simulink model "Squelette_DSPBuilder_ModulateurOQPSK"  (R2016a)
settings: Solver=FixedStepDiscrete  StartTime=0.0  StopTime=1e-3/500  RelTol=1e-3
InitFcn:
  | %% DSPBuilder Start
  | alt_dspbuilder_update_model(bdroot)
  | %% DSPBuilder End
libraries: allblocks_alteradspbuilder2 x84
settings Model: Creator=rhev2401  LastModifiedBy=dufd2703
settings DataIOCC: LimitDataPoints=on  SaveFormat=Array  SignalLoggingSaveFormat=ModelDataLogs
settings DebuggingCC: SolverPrmCheckMsg=warning  MultiTaskDSMMsg=warning  MultiTaskCondExecSysMsg=none
settings HardwareCC: ProdBitPerPointer=32  ProdLargestAtomicFloat=None  ProdIntDivRoundTo=Undefined  ProdEndianess=Unspecified  ProdWordSize=32  ProdHWDeviceType=32-bit Generic
settings ModelReferenceCC: PropagateSignalLabelsOutOfModel=off
settings ConfigComp: CovModelRefEnable=Off  CovSFcnEnable=off

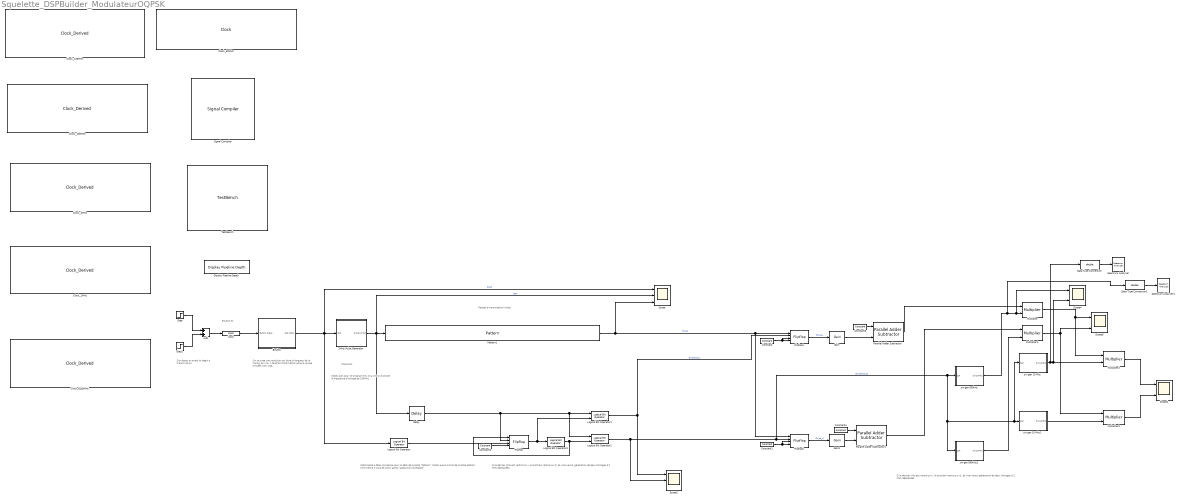
== system Squelette_DSPBuilder_ModulateurOQPSK ==
  note: Simulates an event to begin a transmission
  note: Bouton 01
  note: On se crée une impulsion qui dure la longueur de la trame.
      |
      | En vrai, il faudrait transmettre jusqu'à ce que le buffer soit vide...
  note: Paquet à transmettre (chips)
  note: Chipclock
  note: Notez que, pour ce programme, on a choisi d'utiliser la fréquence d'horloge de 100MHz.
  note: Si le dernier chip est rentré sur I, le prochain rentre sur Q, et vice-versa; génération de deux horloges d'1 MHz déphasées
  note: Cette boîte à délai compense pour le délai de la boîte "Pattern" (notez que la sortie de la boîte pattern commence 1 coup de clock après l'apparition du Enable)
  note: Si le dernier chip est rentré sur I, le prochain rentre sur Q, et vice-versa; génération de deux horloges d'1 MHz déphasées
  2MHz Pulse Generator : Subsystem
  Add : Sum
  Bouton : Subsystem
  Clock_100MHz : allblocks_alteradspbuilder2/Clock_Derived  ClockNumerator=1  ClockDenominator=2  ResetLatency=0  ResetRegisterCascadeDepth=0  SimulationStartCycle=5  PhaseOffset=0  Reset=aclr_100MHz  ResetType=Active Low  Export=off
  Clock_125MHz : allblocks_alteradspbuilder2/Clock_Derived  ClockNumerator=10  ClockDenominator=25  ResetLatency=0  ResetRegisterCascadeDepth=0  SimulationStartCycle=5  PhaseOffset=0  Reset=aclr_125MHz  ResetType=Active Low  Export=off
  Clock_1MHz : allblocks_alteradspbuilder2/Clock_Derived  ClockNumerator=50  ClockDenominator=1  ResetLatency=0  ResetRegisterCascadeDepth=0  SimulationStartCycle=5  PhaseOffset=0  Reset=aclr_1MHz  ResetType=Active Low  Export=off
  Clock_2MHz : allblocks_alteradspbuilder2/Clock_Derived  ClockNumerator=25  ClockDenominator=1  ResetLatency=0  ResetRegisterCascadeDepth=0  SimulationStartCycle=5  PhaseOffset=0  Reset=aclr_2MHz  ResetType=Active Low  Export=off
  Clock_50MHz : allblocks_alteradspbuilder2/Clock  ClockPeriod=20  ClockPeriodUnit=ns  SampleTime=20e-9  ResetLatency=0  ResetRegisterCascadeDepth=0  SimulationStartCycle=5  PhaseOffset=0  Reset=aclr  ResetType=Active Low  Export=off
  Clock_62p5MHz : allblocks_alteradspbuilder2/Clock_Derived  ClockNumerator=800  ClockDenominator=1  ResetLatency=0  ResetRegisterCascadeDepth=0  SimulationStartCycle=5  PhaseOffset=0  Reset=aclr_62p5MHz  ResetType=Active Low  Export=off
  Constant : allblocks_alteradspbuilder2/Constant  mask_cst=1  BusType=Signed Integer  bwl=8  bwr=0  roundMode=Truncate  satMode=Wrap  SpecifyClock=off  allowFloatingPointOverride=on  logOutputs=off  logFile=U:\projet-s6\DSP builder\Squelette_ModulateurOQPSK\tb_Squelette_DSPBuilder_ModulateurOQPSK\Squelette%5FDSPBuilder%5FModulateurOQPSK_Constant.fixedpointlog
  Constant1 : allblocks_alteradspbuilder2/Constant  mask_cst=1  BusType=Signed Integer  bwl=8  bwr=0  roundMode=Truncate  satMode=Wrap  SpecifyClock=off  allowFloatingPointOverride=on  logOutputs=off  logFile=U:\projet-s6\DSP builder\Squelette_ModulateurOQPSK\tb_Squelette_DSPBuilder_ModulateurOQPSK\Squelette%5FDSPBuilder%5FModulateurOQPSK_Constant1.fixedpointlog
  Constant2 : allblocks_alteradspbuilder2/Constant  mask_cst=1  BusType=Signed Integer  bwl=8  bwr=0  roundMode=Truncate  satMode=Wrap  SpecifyClock=off  allowFloatingPointOverride=on  logOutputs=off  logFile=U:\projet-s6\DSP builder\Squelette_ModulateurOQPSK\tb_Squelette_DSPBuilder_ModulateurOQPSK\Squelette%5FDSPBuilder%5FModulateurOQPSK_Constant2.fixedpointlog
  Constant3 : allblocks_alteradspbuilder2/Constant  mask_cst=1  BusType=Unsigned Integer  bwl=1  bwr=0  roundMode=Truncate  satMode=Wrap  SpecifyClock=off  allowFloatingPointOverride=on  logOutputs=off  logFile=U:\projet-s6\DSP builder\Squelette_ModulateurOQPSK\tb_Squelette_DSPBuilder_ModulateurOQPSK\Squelette%5FDSPBuilder%5FModulateurOQPSK_Constant3.fixedpointlog
  Constant4 : allblocks_alteradspbuilder2/Constant  mask_cst=1  BusType=Unsigned Integer  bwl=1  bwr=0  roundMode=Truncate  satMode=Wrap  SpecifyClock=off  allowFloatingPointOverride=on  logOutputs=off  logFile=U:\projet-s6\DSP builder\Squelette_ModulateurOQPSK\tb_Squelette_DSPBuilder_ModulateurOQPSK\Squelette%5FDSPBuilder%5FModulateurOQPSK_Constant4.fixedpointlog
  Data Type Conversion : DataTypeConversion  OutDataTypeStr=double
  Data Type Conversion1 : DataTypeConversion  OutDataTypeStr=double
  Delay : allblocks_alteradspbuilder2/Delay  pipeline=1  pipeline_display=1  ClockPhase=1  use_ena=off  use_sclr=off  allowFloatingPointOverride=on  logOutputs=off  logFile=U:\projet-s6\DSP builder\Squelette_ModulateurOQPSK\tb_Squelette_DSPBuilder_ModulateurOQPSK\Squelette%5FDSPBuilder%5FModulateurOQPSK_Delay.fixedpointlog  use_init=off  reset_value=1
  Display Pipeline Depth : allblocks_alteradspbuilder2/Display Pipeline Depth  DisplayLatencyOnBlocks=on
  Flipflop : allblocks_alteradspbuilder2/Flipflop  mode=DFFE  BusType=Single Bit  bwl=2  bwr=2  pipeline_display=1
  Flipflop1 : allblocks_alteradspbuilder2/Flipflop  mode=DFFE  BusType=Single Bit  bwl=2  bwr=2  pipeline_display=1
  Flipflop2 : allblocks_alteradspbuilder2/Flipflop  mode=DFFE  BusType=Single Bit  bwl=2  bwr=2  pipeline_display=1
  Gain : allblocks_alteradspbuilder2/Gain  vgain=2  BusType=Signed Integer  bwl=3  bwr=0  pipeline=1  pipeline_display=1  allowFloatingPointOverride=on  logOutputs=off  logFile=U:\projet-s6\DSP builder\Squelette_ModulateurOQPSK\tb_Squelette_DSPBuilder_ModulateurOQPSK\Squelette%5FDSPBuilder%5FModulateurOQPSK_Gain.fixedpointlog  use_ena=off  use_aclr=off  lpm=off  MaskValue=1
  Gain1 : allblocks_alteradspbuilder2/Gain  vgain=2  BusType=Signed Integer  bwl=3  bwr=0  pipeline=1  pipeline_display=1  allowFloatingPointOverride=on  logOutputs=off  logFile=U:\projet-s6\DSP builder\Squelette_ModulateurOQPSK\tb_Squelette_DSPBuilder_ModulateurOQPSK\Squelette%5FDSPBuilder%5FModulateurOQPSK_Gain1.fixedpointlog  use_ena=off  use_aclr=off  lpm=off  MaskValue=1
  Input : allblocks_alteradspbuilder2/Input  iofile=U:\projet-s6\DSP builder\Squelette_ModulateurOQPSK\tb_Squelette_DSPBuilder_ModulateurOQPSK\Squelette%5FDSPBuilder%5FModulateurOQPSK_Input.salt  BusType=Single Bit  bwl=1  bwr=0  SpecifyClock=on  clock=Clock_100MHz  PORTTYPE=Input  externalType=Inferred  allowFloatingPointOverride=on  logOutputs=off
  Logical Bit Operator : allblocks_alteradspbuilder2/Logical Bit Operator  LogicalOperator=NOT  user_inputs=2  pipeline_display=0
  Logical Bit Operator1 : allblocks_alteradspbuilder2/Logical Bit Operator  LogicalOperator=AND  user_inputs=2  pipeline_display=0
  Logical Bit Operator2 : allblocks_alteradspbuilder2/Logical Bit Operator  LogicalOperator=AND  user_inputs=2  pipeline_display=0
  Logical Bit Operator3 : allblocks_alteradspbuilder2/Logical Bit Operator  LogicalOperator=NOT  user_inputs=2  pipeline_display=0
  Multiplier : allblocks_alteradspbuilder2/Multiplier  BusType=Signed Integer  bwl=6  bwr=0  pipeline=0  pipeline_display=0  allowFloatingPointOverride=on  logOutputs=off  logFile=U:\projet-s6\DSP builder\Squelette_ModulateurOQPSK\tb_Squelette_DSPBuilder_ModulateurOQPSK\Squelette%5FDSPBuilder%5FModulateurOQPSK_Multiplier.fixedpointlog  UseEqualInputWidth=off  bbwl=14  bbwr=0  FullResolution=on  OutputMsb=8  OutputLsb=0  OutputBwl=16  OutputBwr=16  UseDedicatedCircuitry=YES  use_ena=off  use_aclr=off
  Multiplier1 : allblocks_alteradspbuilder2/Multiplier  BusType=Signed Integer  bwl=6  bwr=0  pipeline=0  pipeline_display=0  allowFloatingPointOverride=on  logOutputs=off  logFile=U:\projet-s6\DSP builder\Squelette_ModulateurOQPSK\tb_Squelette_DSPBuilder_ModulateurOQPSK\Squelette%5FDSPBuilder%5FModulateurOQPSK_Multiplier1.fixedpointlog  UseEqualInputWidth=off  bbwl=14  bbwr=0  FullResolution=on  OutputMsb=8  OutputLsb=0  OutputBwl=16  OutputBwr=16  UseDedicatedCircuitry=YES  use_ena=off  use_aclr=off
  Multiplier2 : allblocks_alteradspbuilder2/Multiplier  BusType=Signed Integer  bwl=16  bwr=0  pipeline=0  pipeline_display=0  allowFloatingPointOverride=on  logOutputs=off  logFile=U:\projet-s6\DSP builder\Squelette_ModulateurOQPSK\tb_Squelette_DSPBuilder_ModulateurOQPSK\Squelette%5FDSPBuilder%5FModulateurOQPSK_Multiplier2.fixedpointlog  UseEqualInputWidth=off  bbwl=14  bbwr=0  FullResolution=on  OutputMsb=8  OutputLsb=0  OutputBwl=16  OutputBwr=16  UseDedicatedCircuitry=YES  use_ena=off  use_aclr=off
  Multiplier3 : allblocks_alteradspbuilder2/Multiplier  BusType=Signed Integer  bwl=16  bwr=0  pipeline=0  pipeline_display=0  allowFloatingPointOverride=on  logOutputs=off  logFile=U:\projet-s6\DSP builder\Squelette_ModulateurOQPSK\tb_Squelette_DSPBuilder_ModulateurOQPSK\Squelette%5FDSPBuilder%5FModulateurOQPSK_Multiplier3.fixedpointlog  UseEqualInputWidth=off  bbwl=14  bbwr=0  FullResolution=on  OutputMsb=8  OutputLsb=0  OutputBwl=16  OutputBwr=16  UseDedicatedCircuitry=YES  use_ena=off  use_aclr=off
  Parallel Adder Subtractor : allblocks_alteradspbuilder2/Parallel Adder Subtractor  number_of_inputs=2  direction=-+  use_pipeline=off  pipeline_display=0  phase_selection=1  use_ena=off  use_aclr=off  allowFloatingPointOverride=on  logOutputs=off  logFile=U:\projet-s6\DSP builder\Squelette_ModulateurOQPSK\tb_Squelette_DSPBuilder_ModulateurOQPSK\Squelette%5FDSPBuilder%5FModulateurOQPSK_Parallel+Adder+Subtractor.fixedpointlog
  Parallel Adder Subtractor1 : allblocks_alteradspbuilder2/Parallel Adder Subtractor  number_of_inputs=2  direction=-+  use_pipeline=off  pipeline_display=0  phase_selection=1  use_ena=off  use_aclr=off  allowFloatingPointOverride=on  logOutputs=off  logFile=U:\projet-s6\DSP builder\Squelette_ModulateurOQPSK\tb_Squelette_DSPBuilder_ModulateurOQPSK\Squelette%5FDSPBuilder%5FModulateurOQPSK_Parallel+Adder+Subtractor1.fixedpointlog
  Pattern1 : allblocks_alteradspbuilder2/Pattern  Sequence=10011010111100001100110000110011  SpecifyClock=off  clock=Clock_250kHz  use_ena=on  use_sclr=off
  Scope : Scope  NumInputPorts=3
  Scope1 : Scope  NumInputPorts=2
  Scope2 : Scope  NumInputPorts=3
  Scope3 : Scope  NumInputPorts=2
  Scope4 : Scope  NumInputPorts=2
  Signal Compiler : allblocks_alteradspbuilder2/Signal Compiler  DeviceFamily=Cyclone V  DeviceName=AUTO  DisableEarlyHDLGeneration=off  EnableSignalTap=off  SignalTapDepth=128  UseBoardBlock=off  StpUseDefaultClock=on  StpClock=Clock_50MHz  ExportDir=C:\Users\pivd2501\Documents  MAX10_ProgrammingMode=Internal Flash (SDM) Single Boot
  Spectrum Analyzer : SpectrumAnalyzer
  Spectrum Analyzer1 : SpectrumAnalyzer
  Step : Step  Time=100e-6  Before=1  After=0  SampleTime=1/100e06  VectorParams1D=off
  Step1 : Step  Time=200e-6  SampleTime=1/100e06  VectorParams1D=off
  TestBench : allblocks_alteradspbuilder2/TestBench  enable=on  advancedMode=on  modelSimGui=on  maxDisplayErrors=1000  mismatchErrorLevel=Error  simdatafile=U:\projet-s6\DSP builder\Squelette_ModulateurOQPSK\tb_Squelette_DSPBuilder_ModulateurOQPSK\Squelette_DSPBuilder_ModulateurOQPSK.simdata.tcl
  sin gen 10 Mhz : Subsystem
  sin gen 10 Mhz1 : Subsystem
  sin gen 500kHz : Subsystem
  sin gen 500kHz2 : Subsystem
  wires:
  Add/1 -> Input/1
  Step1/1 -> Add/2
  Step/1 -> Add/1
  2MHz Pulse Generator/1(Pulse 2MHz) -> Delay/1, Pattern1/1, Scope/2  "ENA"
  Pattern1/1 -> Flipflop2/1, Flipflop1/1, Scope/3  "Chips"
  Bouton/1(CLR 480u) -> Logical Bit Operator/1, 2MHz Pulse Generator/1(CLR), Scope/1  "SCLR"
  Input/1 -> Bouton/1(Button Press)
  Flipflop/1 -> Logical Bit Operator1/2, Logical Bit Operator3/1
  Logical Bit Operator3/1 -> Flipflop/1, Logical Bit Operator2/2
  Logical Bit Operator1/1 -> Scope2/1, Flipflop1/2  "ChipClock_I"
  Constant/1 -> Flipflop1/4, Flipflop1/3
  Constant1/1 -> Flipflop2/3, Flipflop2/4
  Logical Bit Operator2/1 -> Scope2/2, sin gen 10 Mhz/1(CLR), sin gen 10 Mhz1/1(CLR), sin gen 500kHz2/1(CLR), sin gen 500kHz/1(CLR), Flipflop2/2  "ChipClock_Q"
  Logical Bit Operator/1 -> Flipflop/3
  Constant2/1 -> Flipflop/4
  Delay/1 -> Flipflop/2, Logical Bit Operator2/1, Logical Bit Operator1/1
  sin gen 500kHz/1(Sin10Mhz) -> Data Type Conversion1/1, Scope4/1, Multiplier/2
  sin gen 500kHz2/1(Sin10Mhz) -> Multiplier1/2
  Multiplier/1 -> Scope3/1, Multiplier2/1
  Multiplier1/1 -> Multiplier3/1, Scope3/2
  sin gen 10 Mhz/1(Sin10Mhz) -> Data Type Conversion/1, Scope4/2, Multiplier2/2
  sin gen 10 Mhz1/1(Sin10Mhz) -> Multiplier3/2
  Multiplier2/1 -> Scope1/1
  Multiplier3/1 -> Scope1/2
  Flipflop1/1 -> Gain/1  "Chips_I"
  Parallel Adder Subtractor/1 -> Multiplier/1
  Constant3/1 -> Parallel Adder Subtractor/1
  Gain/1 -> Parallel Adder Subtractor/2
  Flipflop2/1 -> Gain1/1  "Chips_Q"
  Gain1/1 -> Parallel Adder Subtractor1/2
  Constant4/1 -> Parallel Adder Subtractor1/1
  Parallel Adder Subtractor1/1 -> Multiplier1/1
  Data Type Conversion/1 -> Spectrum Analyzer/1
  Data Type Conversion1/1 -> Spectrum Analyzer1/1

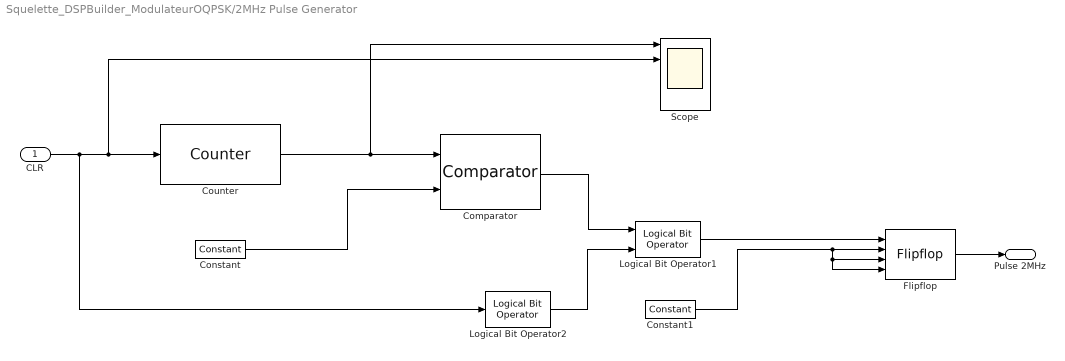
== system Squelette_DSPBuilder_ModulateurOQPSK/2MHz Pulse Generator ==
  CLR : Inport
  Comparator : allblocks_alteradspbuilder2/Comparator  direction=a == b  pipeline_display=0  allowFloatingPointOverride=on  logOutputs=off  logFile=U:\projet-s6\DSP builder\Squelette_ModulateurOQPSK\tb_Squelette_DSPBuilder_ModulateurOQPSK\Squelette%5FDSPBuilder%5FModulateurOQPSK_2MHz+Pulse+Generator_Comparator.fixedpointlog
  Constant : allblocks_alteradspbuilder2/Constant  mask_cst=0  BusType=Unsigned Integer  bwl=1  bwr=0  roundMode=Truncate  satMode=Wrap  SpecifyClock=off  allowFloatingPointOverride=on  logOutputs=off  logFile=U:\projet-s6\DSP builder\Squelette_ModulateurOQPSK\tb_Squelette_DSPBuilder_ModulateurOQPSK\Squelette%5FDSPBuilder%5FModulateurOQPSK_2MHz+Pulse+Generator_Constant.fixedpointlog
  Constant1 : allblocks_alteradspbuilder2/Constant  mask_cst=1  BusType=Unsigned Integer  bwl=1  bwr=0  roundMode=Truncate  satMode=Wrap  SpecifyClock=off  allowFloatingPointOverride=on  logOutputs=off  logFile=U:\projet-s6\DSP builder\Squelette_ModulateurOQPSK\tb_Squelette_DSPBuilder_ModulateurOQPSK\Squelette%5FDSPBuilder%5FModulateurOQPSK_2MHz+Pulse+Generator_Constant1.fixedpointlog
  Counter : allblocks_alteradspbuilder2/Counter  BusType=Unsigned Integer  bwl=10  bwr=0  use_modulo=on  modulo=50  SpecifyClock=off  direction=Increment  use_sload=off  use_sset=off  svalue=1  use_clk_ena=off  use_ena=off  use_sclr=on  pipeline_display=1
  Flipflop : allblocks_alteradspbuilder2/Flipflop  mode=DFFE  BusType=Single Bit  bwl=2  bwr=2  pipeline_display=1
  Logical Bit Operator1 : allblocks_alteradspbuilder2/Logical Bit Operator  LogicalOperator=AND  user_inputs=2  pipeline_display=0
  Logical Bit Operator2 : allblocks_alteradspbuilder2/Logical Bit Operator  LogicalOperator=NOT  user_inputs=2  pipeline_display=0
  Scope : Scope  NumInputPorts=5
  Pulse 2MHz : Outport
  wires:
  Counter/1 -> Scope/1, Comparator/1
  Constant/1 -> Comparator/2
  CLR/1 -> Logical Bit Operator2/1, Scope/2, Counter/1
  Logical Bit Operator2/1 -> Logical Bit Operator1/2
  Comparator/1 -> Logical Bit Operator1/1
  Flipflop/1 -> Pulse 2MHz/1
  Logical Bit Operator1/1 -> Flipflop/1
  Constant1/1 -> Flipflop/4, Flipflop/3, Flipflop/2

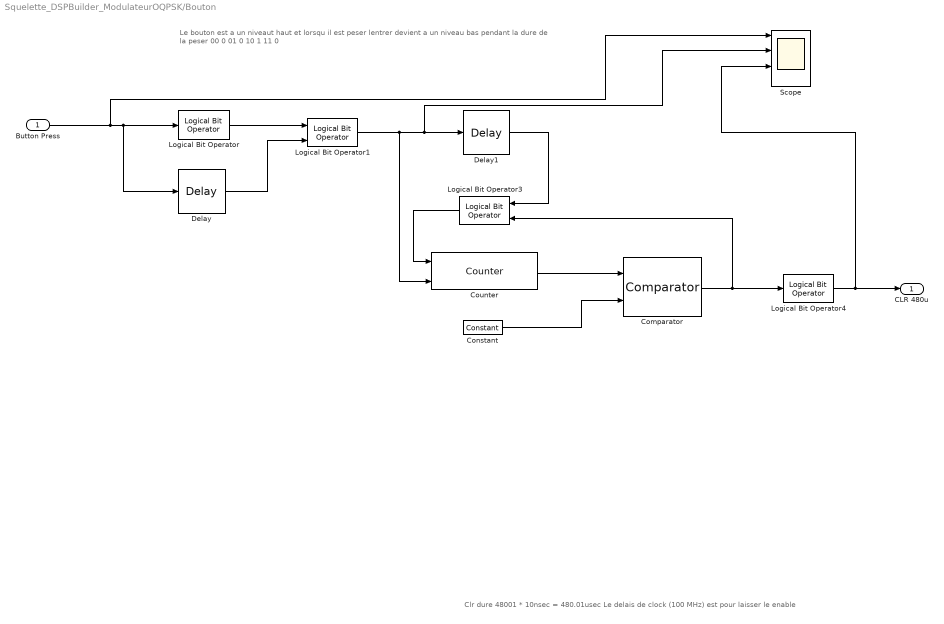
== system Squelette_DSPBuilder_ModulateurOQPSK/Bouton ==
  note: Clr dure 48001 * 10nsec = 480.01usec Le delais de clock (100 MHz) est pour laisser le enable
  note: Le bouton est a un niveaut haut et lorsqu il est peser lentrer devient a un niveau bas pendant la dure de la peser
      |
      | 00  0
      | 01  0
      | 10  1
      | 11  0
  Button Press : Inport
  Comparator : allblocks_alteradspbuilder2/Comparator  direction=a >= b  pipeline_display=0  allowFloatingPointOverride=on  logOutputs=off  logFile=U:\projet-s6\DSP builder\Squelette_ModulateurOQPSK\tb_Squelette_DSPBuilder_ModulateurOQPSK\Squelette%5FDSPBuilder%5FModulateurOQPSK_Bouton_Comparator.fixedpointlog
  Constant : allblocks_alteradspbuilder2/Constant  mask_cst=1  BusType=Unsigned Integer  bwl=8  bwr=0  roundMode=Truncate  satMode=Wrap  SpecifyClock=off  allowFloatingPointOverride=on  logOutputs=off  logFile=U:\projet-s6\DSP builder\Squelette_ModulateurOQPSK\tb_Squelette_DSPBuilder_ModulateurOQPSK\Squelette%5FDSPBuilder%5FModulateurOQPSK_Bouton_Constant.fixedpointlog
  Counter : allblocks_alteradspbuilder2/Counter  BusType=Unsigned Integer  bwl=16  bwr=0  use_modulo=on  modulo=48001  SpecifyClock=off  clock=Clock_100MHz  direction=Increment  use_sload=off  use_sset=off  svalue=1  use_clk_ena=off  use_ena=on  use_sclr=on  pipeline_display=1
  Delay : allblocks_alteradspbuilder2/Delay  pipeline=1  pipeline_display=1  ClockPhase=1  use_ena=off  use_sclr=off  allowFloatingPointOverride=on  logOutputs=off  logFile=U:\projet-s6\DSP builder\Squelette_ModulateurOQPSK\tb_Squelette_DSPBuilder_ModulateurOQPSK\Squelette%5FDSPBuilder%5FModulateurOQPSK_Bouton_Delay.fixedpointlog  use_init=off  reset_value=1
  Delay1 : allblocks_alteradspbuilder2/Delay  pipeline=1  pipeline_display=1  ClockPhase=1  use_ena=off  use_sclr=off  allowFloatingPointOverride=on  logOutputs=off  logFile=U:\projet-s6\DSP builder\Squelette_ModulateurOQPSK\tb_Squelette_DSPBuilder_ModulateurOQPSK\Squelette%5FDSPBuilder%5FModulateurOQPSK_Bouton_Delay1.fixedpointlog  use_init=off  reset_value=1
  Logical Bit Operator : allblocks_alteradspbuilder2/Logical Bit Operator  LogicalOperator=NOT  user_inputs=2  pipeline_display=0
  Logical Bit Operator1 : allblocks_alteradspbuilder2/Logical Bit Operator  LogicalOperator=AND  user_inputs=2  pipeline_display=0
  Logical Bit Operator3 : allblocks_alteradspbuilder2/Logical Bit Operator  LogicalOperator=OR  user_inputs=2  pipeline_display=0
  Logical Bit Operator4 : allblocks_alteradspbuilder2/Logical Bit Operator  LogicalOperator=NOT  user_inputs=2  pipeline_display=0
  Scope : Scope  NumInputPorts=4
  CLR 480u : Outport
  wires:
  Button Press/1 -> Scope/1, Logical Bit Operator/1, Delay/1
  Logical Bit Operator/1 -> Logical Bit Operator1/1
  Logical Bit Operator1/1 -> Scope/2, Delay1/1, Counter/2
  Counter/1 -> Comparator/1
  Constant/1 -> Comparator/2
  Delay1/1 -> Logical Bit Operator3/1
  Logical Bit Operator3/1 -> Counter/1
  Comparator/1 -> Logical Bit Operator3/2, Logical Bit Operator4/1
  Delay/1 -> Logical Bit Operator1/2
  Logical Bit Operator4/1 -> Scope/3, CLR 480u/1

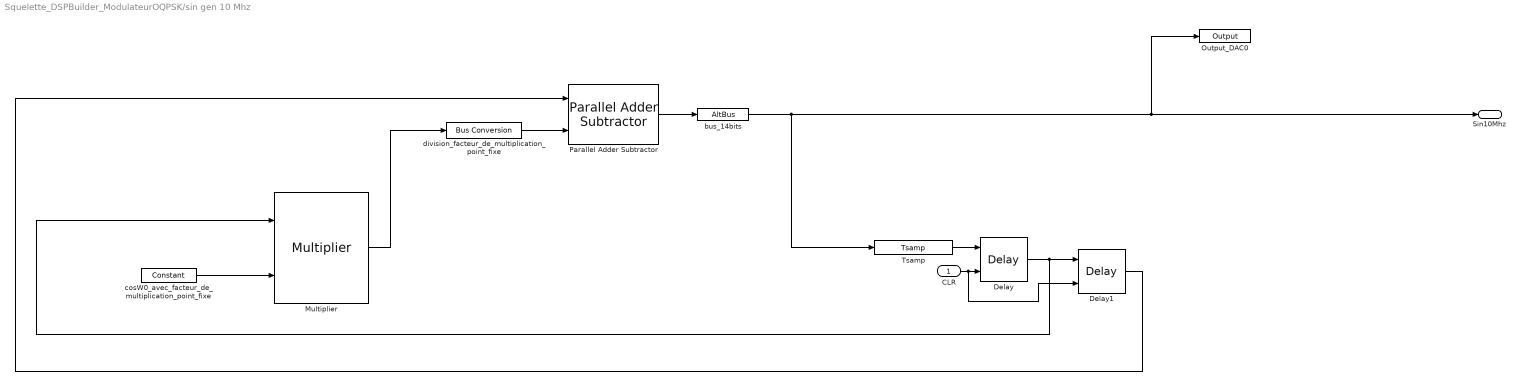
== system Squelette_DSPBuilder_ModulateurOQPSK/sin gen 10 Mhz ==
  CLR : Inport
  Delay : allblocks_alteradspbuilder2/Delay  pipeline=1  pipeline_display=1  ClockPhase=1  use_ena=off  use_sclr=on  allowFloatingPointOverride=on  logOutputs=off  logFile=U:\projet-s6\DSP builder\Squelette_ModulateurOQPSK\tb_Squelette_DSPBuilder_ModulateurOQPSK\Squelette%5FDSPBuilder%5FModulateurOQPSK_sin+gen+10+Mhz_Delay.fixedpointlog  use_init=on  reset_value=y_n_1_10M
  Delay1 : allblocks_alteradspbuilder2/Delay  pipeline=1  pipeline_display=1  ClockPhase=1  use_ena=off  use_sclr=on  allowFloatingPointOverride=on  logOutputs=off  logFile=U:\projet-s6\DSP builder\Squelette_ModulateurOQPSK\tb_Squelette_DSPBuilder_ModulateurOQPSK\Squelette%5FDSPBuilder%5FModulateurOQPSK_sin+gen+10+Mhz_Delay1.fixedpointlog  use_init=on  reset_value=y_n_2_10M
  Multiplier : allblocks_alteradspbuilder2/Multiplier  BusType=Signed Integer  bwl=14  bwr=0  pipeline=0  pipeline_display=0  allowFloatingPointOverride=on  logOutputs=off  logFile=U:\projet-s6\DSP builder\Squelette_ModulateurOQPSK\tb_Squelette_DSPBuilder_ModulateurOQPSK\Squelette%5FDSPBuilder%5FModulateurOQPSK_sin+gen+10+Mhz_Multiplier.fixedpointlog  UseEqualInputWidth=off  bbwl=19  bbwr=0  FullResolution=on  OutputMsb=8  OutputLsb=0  OutputBwl=16  OutputBwr=16  UseDedicatedCircuitry=YES  use_ena=off  use_aclr=off
  Output_DAC0 : allblocks_alteradspbuilder2/Output  iofile=U:\projet-s6\DSP builder\Squelette_ModulateurOQPSK\tb_Squelette_DSPBuilder_ModulateurOQPSK\Squelette%5FDSPBuilder%5FModulateurOQPSK_sin+gen+10+Mhz_Output%5FDAC0.capture  BusType=Signed Integer  bwl=14  bwr=0  externalType=Inferred  PORTTYPE=Output  allowFloatingPointOverride=on  logOutputs=off
  Parallel Adder Subtractor : allblocks_alteradspbuilder2/Parallel Adder Subtractor  number_of_inputs=2  direction=-+  use_pipeline=off  pipeline_display=0  phase_selection=1  use_ena=off  use_aclr=off  allowFloatingPointOverride=on  logOutputs=off  logFile=U:\projet-s6\DSP builder\Squelette_ModulateurOQPSK\tb_Squelette_DSPBuilder_ModulateurOQPSK\Squelette%5FDSPBuilder%5FModulateurOQPSK_sin+gen+10+Mhz_Parallel+Adder+Subtractor.fixedpointlog
  Tsamp : allblocks_alteradspbuilder2/Tsamp  SpecifyClock=on  clock=Clock_100MHz
  bus_14bits : allblocks_alteradspbuilder2/AltBus  BusType=Signed Integer  bwl=14  bwr=0  saturate=off  floatingPointInput=on  floatingPointOutput=on  logOutputs=off  logFile=U:\projet-s6\DSP builder\Squelette_ModulateurOQPSK\tb_Squelette_DSPBuilder_ModulateurOQPSK\Squelette%5FDSPBuilder%5FModulateurOQPSK_sin+gen+10+Mhz_bus%5F14bits.fixedpointlog
  cosW0_avec_facteur_de_multiplication_point_fixe : allblocks_alteradspbuilder2/Constant  mask_cst=a1_10M  BusType=Signed Integer  bwl=19  bwr=0  roundMode=Truncate  satMode=Wrap  SpecifyClock=off  allowFloatingPointOverride=on  logOutputs=off  logFile=U:\projet-s6\DSP builder\Squelette_ModulateurOQPSK\tb_Squelette_DSPBuilder_ModulateurOQPSK\Squelette%5FDSPBuilder%5FModulateurOQPSK_sin+gen+10+Mhz_cosW0%5Favec%5Ffacteur%5Fde%5Fmultiplication%5Fpoint%5Ffixe.fixedpointlog
  division_facteur_de_multiplication_point_fixe : allblocks_alteradspbuilder2/Bus Conversion  BusType=Signed Integer  ibwl=33  ibwr=1  bwl=14  bwr=1  bitToConnectToOutputLSB=16  round=off  saturate=off  pipeline_display=0
  Sin10Mhz : Outport
  wires:
  Delay/1 -> Multiplier/1, Delay1/1
  cosW0_avec_facteur_de_multiplication_point_fixe/1 -> Multiplier/2
  Delay1/1 -> Parallel Adder Subtractor/1
  bus_14bits/1 -> Sin10Mhz/1, Output_DAC0/1, Tsamp/1
  Parallel Adder Subtractor/1 -> bus_14bits/1
  division_facteur_de_multiplication_point_fixe/1 -> Parallel Adder Subtractor/2
  Multiplier/1 -> division_facteur_de_multiplication_point_fixe/1
  Tsamp/1 -> Delay/1
  CLR/1 -> Delay1/2, Delay/2

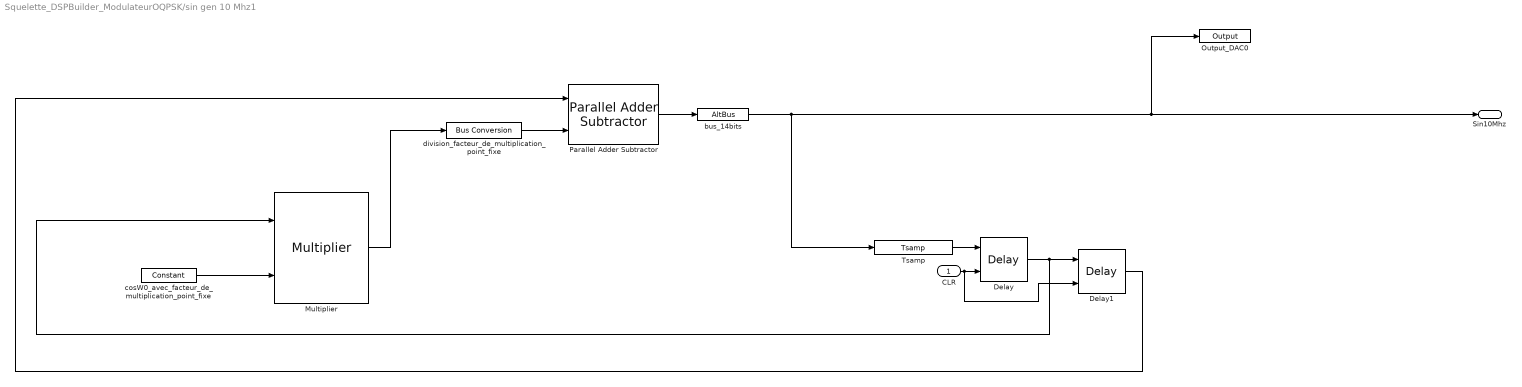
== system Squelette_DSPBuilder_ModulateurOQPSK/sin gen 10 Mhz1 ==
  CLR : Inport
  Delay : allblocks_alteradspbuilder2/Delay  pipeline=1  pipeline_display=1  ClockPhase=1  use_ena=off  use_sclr=on  allowFloatingPointOverride=on  logOutputs=off  logFile=U:\projet-s6\DSP builder\Squelette_ModulateurOQPSK\tb_Squelette_DSPBuilder_ModulateurOQPSK\Squelette%5FDSPBuilder%5FModulateurOQPSK_sin+gen+10+Mhz1_Delay.fixedpointlog  use_init=on  reset_value=y_n_1_10M
  Delay1 : allblocks_alteradspbuilder2/Delay  pipeline=1  pipeline_display=1  ClockPhase=1  use_ena=off  use_sclr=on  allowFloatingPointOverride=on  logOutputs=off  logFile=U:\projet-s6\DSP builder\Squelette_ModulateurOQPSK\tb_Squelette_DSPBuilder_ModulateurOQPSK\Squelette%5FDSPBuilder%5FModulateurOQPSK_sin+gen+10+Mhz1_Delay1.fixedpointlog  use_init=on  reset_value=y_n_2_10M
  Multiplier : allblocks_alteradspbuilder2/Multiplier  BusType=Signed Integer  bwl=14  bwr=0  pipeline=0  pipeline_display=0  allowFloatingPointOverride=on  logOutputs=off  logFile=U:\projet-s6\DSP builder\Squelette_ModulateurOQPSK\tb_Squelette_DSPBuilder_ModulateurOQPSK\Squelette%5FDSPBuilder%5FModulateurOQPSK_sin+gen+10+Mhz1_Multiplier.fixedpointlog  UseEqualInputWidth=off  bbwl=19  bbwr=0  FullResolution=on  OutputMsb=8  OutputLsb=0  OutputBwl=16  OutputBwr=16  UseDedicatedCircuitry=YES  use_ena=off  use_aclr=off
  Output_DAC0 : allblocks_alteradspbuilder2/Output  iofile=U:\projet-s6\DSP builder\Squelette_ModulateurOQPSK\tb_Squelette_DSPBuilder_ModulateurOQPSK\Squelette%5FDSPBuilder%5FModulateurOQPSK_sin+gen+10+Mhz1_Output%5FDAC0.capture  BusType=Signed Integer  bwl=14  bwr=0  externalType=Inferred  PORTTYPE=Output  allowFloatingPointOverride=on  logOutputs=off
  Parallel Adder Subtractor : allblocks_alteradspbuilder2/Parallel Adder Subtractor  number_of_inputs=2  direction=-+  use_pipeline=off  pipeline_display=0  phase_selection=1  use_ena=off  use_aclr=off  allowFloatingPointOverride=on  logOutputs=off  logFile=U:\projet-s6\DSP builder\Squelette_ModulateurOQPSK\tb_Squelette_DSPBuilder_ModulateurOQPSK\Squelette%5FDSPBuilder%5FModulateurOQPSK_sin+gen+10+Mhz1_Parallel+Adder+Subtractor.fixedpointlog
  Tsamp : allblocks_alteradspbuilder2/Tsamp  SpecifyClock=on  clock=Clock_100MHz
  bus_14bits : allblocks_alteradspbuilder2/AltBus  BusType=Signed Integer  bwl=14  bwr=0  saturate=off  floatingPointInput=on  floatingPointOutput=on  logOutputs=off  logFile=U:\projet-s6\DSP builder\Squelette_ModulateurOQPSK\tb_Squelette_DSPBuilder_ModulateurOQPSK\Squelette%5FDSPBuilder%5FModulateurOQPSK_sin+gen+10+Mhz1_bus%5F14bits.fixedpointlog
  cosW0_avec_facteur_de_multiplication_point_fixe : allblocks_alteradspbuilder2/Constant  mask_cst=a1_10M  BusType=Signed Integer  bwl=19  bwr=0  roundMode=Truncate  satMode=Wrap  SpecifyClock=off  allowFloatingPointOverride=on  logOutputs=off  logFile=U:\projet-s6\DSP builder\Squelette_ModulateurOQPSK\tb_Squelette_DSPBuilder_ModulateurOQPSK\Squelette%5FDSPBuilder%5FModulateurOQPSK_sin+gen+10+Mhz1_cosW0%5Favec%5Ffacteur%5Fde%5Fmultiplication%5Fpoint%5Ffixe.fixedpointlog
  division_facteur_de_multiplication_point_fixe : allblocks_alteradspbuilder2/Bus Conversion  BusType=Signed Integer  ibwl=33  ibwr=1  bwl=14  bwr=1  bitToConnectToOutputLSB=16  round=off  saturate=off  pipeline_display=0
  Sin10Mhz : Outport
  wires:
  CLR/1 -> Delay1/2, Delay/2
  Tsamp/1 -> Delay/1
  Multiplier/1 -> division_facteur_de_multiplication_point_fixe/1
  division_facteur_de_multiplication_point_fixe/1 -> Parallel Adder Subtractor/2
  Parallel Adder Subtractor/1 -> bus_14bits/1
  bus_14bits/1 -> Tsamp/1, Output_DAC0/1, Sin10Mhz/1
  Delay1/1 -> Parallel Adder Subtractor/1
  cosW0_avec_facteur_de_multiplication_point_fixe/1 -> Multiplier/2
  Delay/1 -> Delay1/1, Multiplier/1

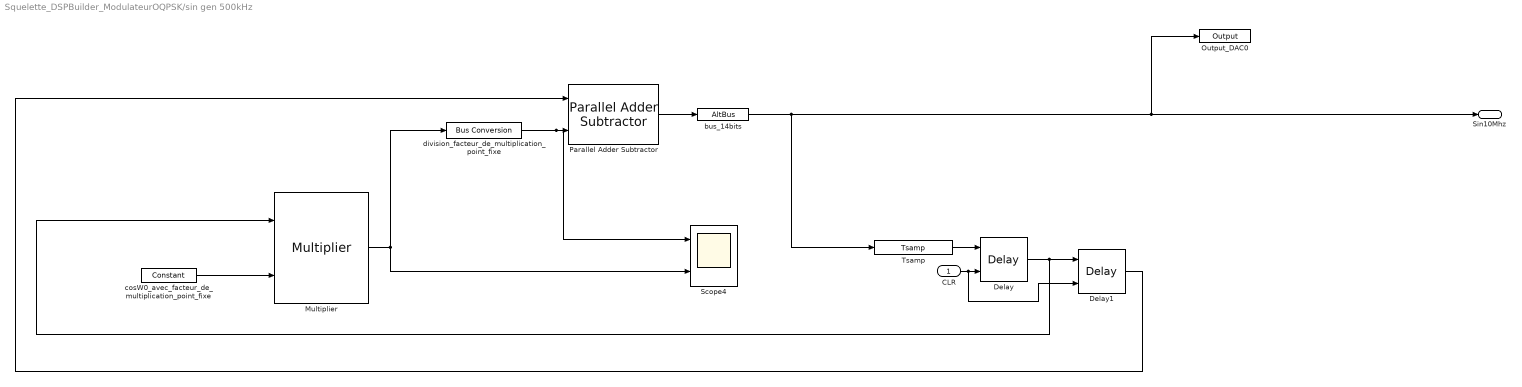
== system Squelette_DSPBuilder_ModulateurOQPSK/sin gen 500kHz ==
  CLR : Inport
  Delay : allblocks_alteradspbuilder2/Delay  pipeline=1  pipeline_display=1  ClockPhase=1  use_ena=off  use_sclr=on  allowFloatingPointOverride=on  logOutputs=off  logFile=U:\projet-s6\DSP builder\Squelette_ModulateurOQPSK\tb_Squelette_DSPBuilder_ModulateurOQPSK\Squelette%5FDSPBuilder%5FModulateurOQPSK_sin+gen+500kHz_Delay.fixedpointlog  use_init=on  reset_value=y_n_1_500k
  Delay1 : allblocks_alteradspbuilder2/Delay  pipeline=1  pipeline_display=1  ClockPhase=1  use_ena=off  use_sclr=on  allowFloatingPointOverride=on  logOutputs=off  logFile=U:\projet-s6\DSP builder\Squelette_ModulateurOQPSK\tb_Squelette_DSPBuilder_ModulateurOQPSK\Squelette%5FDSPBuilder%5FModulateurOQPSK_sin+gen+500kHz_Delay1.fixedpointlog  use_init=on  reset_value=y_n_2_500k
  Multiplier : allblocks_alteradspbuilder2/Multiplier  BusType=Signed Integer  bwl=14  bwr=0  pipeline=0  pipeline_display=0  allowFloatingPointOverride=on  logOutputs=off  logFile=U:\projet-s6\DSP builder\Squelette_ModulateurOQPSK\tb_Squelette_DSPBuilder_ModulateurOQPSK\Squelette%5FDSPBuilder%5FModulateurOQPSK_sin+gen+500kHz_Multiplier.fixedpointlog  UseEqualInputWidth=off  bbwl=19  bbwr=0  FullResolution=on  OutputMsb=8  OutputLsb=0  OutputBwl=16  OutputBwr=16  UseDedicatedCircuitry=YES  use_ena=off  use_aclr=off
  Output_DAC0 : allblocks_alteradspbuilder2/Output  iofile=U:\projet-s6\DSP builder\Squelette_ModulateurOQPSK\tb_Squelette_DSPBuilder_ModulateurOQPSK\Squelette%5FDSPBuilder%5FModulateurOQPSK_sin+gen+500kHz_Output%5FDAC0.capture  BusType=Signed Integer  bwl=14  bwr=0  externalType=Inferred  PORTTYPE=Output  allowFloatingPointOverride=on  logOutputs=off
  Parallel Adder Subtractor : allblocks_alteradspbuilder2/Parallel Adder Subtractor  number_of_inputs=2  direction=-+  use_pipeline=off  pipeline_display=0  phase_selection=1  use_ena=off  use_aclr=off  allowFloatingPointOverride=on  logOutputs=off  logFile=U:\projet-s6\DSP builder\Squelette_ModulateurOQPSK\tb_Squelette_DSPBuilder_ModulateurOQPSK\Squelette%5FDSPBuilder%5FModulateurOQPSK_sin+gen+500kHz_Parallel+Adder+Subtractor.fixedpointlog
  Scope4 : Scope  NumInputPorts=2
  Tsamp : allblocks_alteradspbuilder2/Tsamp  SpecifyClock=on  clock=Clock_100MHz
  bus_14bits : allblocks_alteradspbuilder2/AltBus  BusType=Signed Integer  bwl=14  bwr=0  saturate=off  floatingPointInput=on  floatingPointOutput=on  logOutputs=off  logFile=U:\projet-s6\DSP builder\Squelette_ModulateurOQPSK\tb_Squelette_DSPBuilder_ModulateurOQPSK\Squelette%5FDSPBuilder%5FModulateurOQPSK_sin+gen+500kHz_bus%5F14bits.fixedpointlog
  cosW0_avec_facteur_de_multiplication_point_fixe : allblocks_alteradspbuilder2/Constant  mask_cst=a1_500k  BusType=Signed Integer  bwl=19  bwr=0  roundMode=Truncate  satMode=Wrap  SpecifyClock=off  allowFloatingPointOverride=on  logOutputs=off  logFile=U:\projet-s6\DSP builder\Squelette_ModulateurOQPSK\tb_Squelette_DSPBuilder_ModulateurOQPSK\Squelette%5FDSPBuilder%5FModulateurOQPSK_sin+gen+500kHz_cosW0%5Favec%5Ffacteur%5Fde%5Fmultiplication%5Fpoint%5Ffixe.fixedpointlog
  division_facteur_de_multiplication_point_fixe : allblocks_alteradspbuilder2/Bus Conversion  BusType=Signed Integer  ibwl=33  ibwr=1  bwl=14  bwr=1  bitToConnectToOutputLSB=16  round=off  saturate=off  pipeline_display=0
  Sin10Mhz : Outport
  wires:
  CLR/1 -> Delay1/2, Delay/2
  Tsamp/1 -> Delay/1
  Multiplier/1 -> division_facteur_de_multiplication_point_fixe/1, Scope4/2
  division_facteur_de_multiplication_point_fixe/1 -> Scope4/1, Parallel Adder Subtractor/2
  Parallel Adder Subtractor/1 -> bus_14bits/1
  bus_14bits/1 -> Tsamp/1, Output_DAC0/1, Sin10Mhz/1
  Delay1/1 -> Parallel Adder Subtractor/1
  cosW0_avec_facteur_de_multiplication_point_fixe/1 -> Multiplier/2
  Delay/1 -> Delay1/1, Multiplier/1

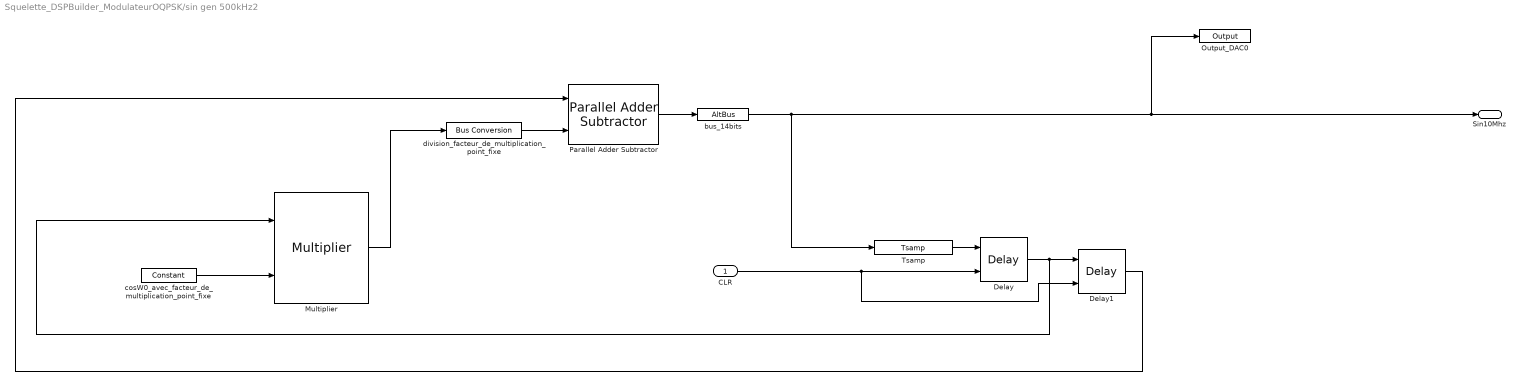
== system Squelette_DSPBuilder_ModulateurOQPSK/sin gen 500kHz2 ==
  CLR : Inport
  Delay : allblocks_alteradspbuilder2/Delay  pipeline=1  pipeline_display=1  ClockPhase=1  use_ena=off  use_sclr=on  allowFloatingPointOverride=on  logOutputs=off  logFile=U:\projet-s6\DSP builder\Squelette_ModulateurOQPSK\tb_Squelette_DSPBuilder_ModulateurOQPSK\Squelette%5FDSPBuilder%5FModulateurOQPSK_sin+gen+500kHz2_Delay.fixedpointlog  use_init=on  reset_value=y_n_1_500k
  Delay1 : allblocks_alteradspbuilder2/Delay  pipeline=1  pipeline_display=1  ClockPhase=1  use_ena=off  use_sclr=on  allowFloatingPointOverride=on  logOutputs=off  logFile=U:\projet-s6\DSP builder\Squelette_ModulateurOQPSK\tb_Squelette_DSPBuilder_ModulateurOQPSK\Squelette%5FDSPBuilder%5FModulateurOQPSK_sin+gen+500kHz2_Delay1.fixedpointlog  use_init=on  reset_value=y_n_2_500k
  Multiplier : allblocks_alteradspbuilder2/Multiplier  BusType=Signed Integer  bwl=14  bwr=0  pipeline=0  pipeline_display=0  allowFloatingPointOverride=on  logOutputs=off  logFile=U:\projet-s6\DSP builder\Squelette_ModulateurOQPSK\tb_Squelette_DSPBuilder_ModulateurOQPSK\Squelette%5FDSPBuilder%5FModulateurOQPSK_sin+gen+500kHz2_Multiplier.fixedpointlog  UseEqualInputWidth=off  bbwl=19  bbwr=0  FullResolution=on  OutputMsb=8  OutputLsb=0  OutputBwl=16  OutputBwr=16  UseDedicatedCircuitry=YES  use_ena=off  use_aclr=off
  Output_DAC0 : allblocks_alteradspbuilder2/Output  iofile=U:\projet-s6\DSP builder\Squelette_ModulateurOQPSK\tb_Squelette_DSPBuilder_ModulateurOQPSK\Squelette%5FDSPBuilder%5FModulateurOQPSK_sin+gen+500kHz2_Output%5FDAC0.capture  BusType=Signed Integer  bwl=14  bwr=0  externalType=Inferred  PORTTYPE=Output  allowFloatingPointOverride=on  logOutputs=off
  Parallel Adder Subtractor : allblocks_alteradspbuilder2/Parallel Adder Subtractor  number_of_inputs=2  direction=-+  use_pipeline=off  pipeline_display=0  phase_selection=1  use_ena=off  use_aclr=off  allowFloatingPointOverride=on  logOutputs=off  logFile=U:\projet-s6\DSP builder\Squelette_ModulateurOQPSK\tb_Squelette_DSPBuilder_ModulateurOQPSK\Squelette%5FDSPBuilder%5FModulateurOQPSK_sin+gen+500kHz2_Parallel+Adder+Subtractor.fixedpointlog
  Tsamp : allblocks_alteradspbuilder2/Tsamp  SpecifyClock=on  clock=Clock_100MHz
  bus_14bits : allblocks_alteradspbuilder2/AltBus  BusType=Signed Integer  bwl=14  bwr=0  saturate=off  floatingPointInput=on  floatingPointOutput=on  logOutputs=off  logFile=U:\projet-s6\DSP builder\Squelette_ModulateurOQPSK\tb_Squelette_DSPBuilder_ModulateurOQPSK\Squelette%5FDSPBuilder%5FModulateurOQPSK_sin+gen+500kHz2_bus%5F14bits.fixedpointlog
  cosW0_avec_facteur_de_multiplication_point_fixe : allblocks_alteradspbuilder2/Constant  mask_cst=a1_500k  BusType=Signed Integer  bwl=19  bwr=0  roundMode=Truncate  satMode=Wrap  SpecifyClock=off  allowFloatingPointOverride=on  logOutputs=off  logFile=U:\projet-s6\DSP builder\Squelette_ModulateurOQPSK\tb_Squelette_DSPBuilder_ModulateurOQPSK\Squelette%5FDSPBuilder%5FModulateurOQPSK_sin+gen+500kHz2_cosW0%5Favec%5Ffacteur%5Fde%5Fmultiplication%5Fpoint%5Ffixe.fixedpointlog
  division_facteur_de_multiplication_point_fixe : allblocks_alteradspbuilder2/Bus Conversion  BusType=Signed Integer  ibwl=33  ibwr=1  bwl=14  bwr=1  bitToConnectToOutputLSB=16  round=off  saturate=off  pipeline_display=0
  Sin10Mhz : Outport
  wires:
  Delay/1 -> Multiplier/1, Delay1/1
  cosW0_avec_facteur_de_multiplication_point_fixe/1 -> Multiplier/2
  Delay1/1 -> Parallel Adder Subtractor/1
  bus_14bits/1 -> Sin10Mhz/1, Output_DAC0/1, Tsamp/1
  Parallel Adder Subtractor/1 -> bus_14bits/1
  division_facteur_de_multiplication_point_fixe/1 -> Parallel Adder Subtractor/2
  Multiplier/1 -> division_facteur_de_multiplication_point_fixe/1
  Tsamp/1 -> Delay/1
  CLR/1 -> Delay1/2, Delay/2
